simulink model "testFrame_PositionObserever"  (R2020b)
settings: Solver=FixedStepDiscrete  StartTime=0.0  StopTime=2  FixedStep=50e-6  RelTol=1e-3
undefined symbols (not defined in the file): BrkPoints, d_q_Voltage_Limiter_sat_neg, d_q_Voltage_Limiter_sat_pos, Ts
libraries: mcbcontrolslib x7, pid_lib x2, simulink x1
settings Model: DataDictionary=MotorControl.sldd  NumberOfSteps=10  Creator=unix  LastModifiedBy=unix
settings DebuggingCC: IntegerOverflowMsg=error  ParameterUnderflowMsg=error  IntegerSaturationMsg=error

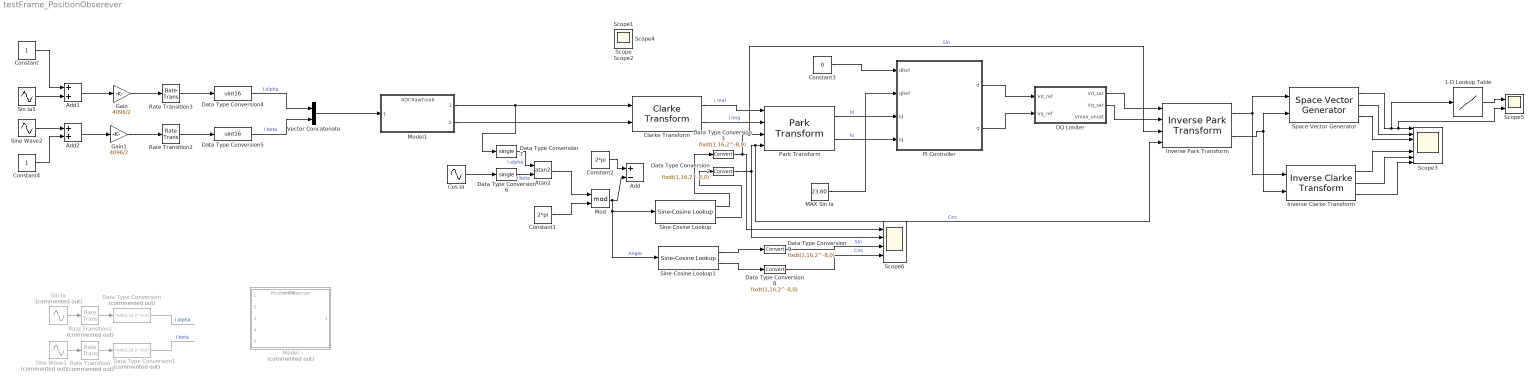
== system testFrame_PositionObserever ==
  1-D Lookup Table : Lookup_n-D  NumberOfTableDimensions=1  BreakpointsForDimension1=BrkPoints  Table=[0 250 500]  ExtrapMethod=Clip  InternalRulePriority=Speed  OutDataTypeStr=uint16  RndMeth=Simplest  SaturateOnIntegerOverflow=on  InputSameDT=on
  Add : Sum  Inputs=+-
  Add1 : Sum
  Add2 : Sum
  Atan2 : Trigonometry  Operator=atan2
  Clarke Transform : mcbcontrolslib/Clarke Transform  VariantControl=Variant2
  Constant : Constant
  Constant1 : Constant  Value=2*pi  OutDataTypeStr=Inherit: Inherit via back propagation
  Constant2 : Constant  Value=2*pi  OutDataTypeStr=Inherit: Inherit via back propagation
  Constant3 : Constant  Value=0  OutDataTypeStr=int8
  Constant4 : Constant
  Cos Ia : Sin  Amplitude=23.6  Frequency=100  Phase=pi/2  SampleTime=0
  DQ Limiter : Subsystem  AncestorBlock=mcbcontrolslib/DQ Limiter  mask(DQ Limiter){Vmax=5}
      mask prompts: Vmax "D-Q saturation limit:"
      mask help:
      | Implement saturation on reference dq voltages, with respect to phase voltage peak limit.
      |
      | The block accepts reference values of d and q axis voltages, and outputs corresponding saturated values along with unsaturated peak value to initiate field weakening control.
      |
      | Enter the phase voltage peak limit in the dialog box to initiate saturation.
      mask Help: eval('mcb.internal.helpview(''dqlimiter'')')
      mask Display: mcb.internal.drawIcons('DQ Limiter',1);
  Data Type Conversion : DataTypeConversion  Commented=on  OutDataTypeStr=fixdt(1,16,2^-8,0)
  Data Type Conversion1 : DataTypeConversion  Commented=on  OutDataTypeStr=fixdt(1,16,2^-8,0)
  Data Type Conversion{2..3,8..9} (4 alike) : DataTypeConversion  OutDataTypeStr=fixdt(1,16,2^-8,0)
  Data Type Conversion4 : DataTypeConversion  OutDataTypeStr=uint16
  Data Type Conversion5 : DataTypeConversion  OutDataTypeStr=uint16
  Data Type Conversion6 : DataTypeConversion  OutDataTypeStr=single
  Data Type Conversion7 : DataTypeConversion  OutDataTypeStr=single
  Gain : Gain  Gain=4096/2
  Gain1 : Gain  Gain=4096/2
  Inverse Clarke Transform : mcbcontrolslib/Inverse Clarke Transform
      settings: SourceProductBaseCode=MT
  Inverse Park Transform : mcbcontrolslib/Inverse Park Transform  AxisAlignment=D-axis
  MAX Sin Ia : Constant  Value=23.60  OutDataTypeStr=Inherit: Inherit via back propagation
  Mod : Math  Operator=mod  SaturateOnIntegerOverflow=on
  Model : ModelReference  Commented=on  ModelNameDialog=PositionObserver.slx  ModelReferenceVersion=3.3  EnablePortName=Enable  EnablePortStatesWhenEnabling=reset
  Model1 : ModelReference  ModelNameDialog=ADCRawToIab.slx  ModelReferenceVersion=3.3
  PI Controller : Subsystem
  Park Transform : mcbcontrolslib/Park Transform  AxisAlignment=D-axis
      settings: SourceProductBaseCode=MT
  Rate Transition : RateTransition  Commented=on  OutPortSampleTime=250e-6
  Rate Transition1 : RateTransition  Commented=on  OutPortSampleTime=250e-6
  Rate Transition2 : RateTransition  OutPortSampleTime=250e-6
  Rate Transition3 : RateTransition  OutPortSampleTime=250e-6
  Scope3 : Scope  NumInputPorts=7
  Scope5 : Scope  NumInputPorts=2
  Scope6 : Scope  NumInputPorts=4
  Sin Ia : Sin  Commented=on  Amplitude=25  Frequency=100  SampleTime=0
  Sin Ia1 : Sin  Frequency=100  SampleTime=0
  Sine Wave1 : Sin  Commented=on  Amplitude=25  Frequency=100  Phase=(2*pi)/3  SampleTime=0
  Sine Wave2 : Sin  Frequency=100  Phase=(2*pi)/3  SampleTime=0
  Sine-Cosine Lookup : mcbcontrolslib/Sine-Cosine Lookup  AngleInput=Radians  N_points=512
      settings: SourceProductBaseCode=MT
  Sine-Cosine Lookup1 : mcbcontrolslib/Sine-Cosine Lookup  AngleInput=Radians  N_points=512
      settings: SourceProductBaseCode=MT
  Space Vector Generator : mcbcontrolslib/Space Vector Generator
      settings: SourceProductBaseCode=MT
  Vector Concatenate : Concatenate
  Scope{,1..2,4} (4 alike) : Scope
  wires:
  Sine-Cosine Lookup/2 -> Data Type Conversion2/1
  Sine-Cosine Lookup/1 -> Data Type Conversion3/1
  Clarke Transform/1 -> Park Transform/1  "I real"
  Clarke Transform/2 -> Park Transform/2  "I img"
  Constant1/1 -> Mod/2
  Park Transform/1 -> PI Controller/3(Id)  "Id"
  Park Transform/2 -> PI Controller/4(Iq)  "Iq"
  Data Type Conversion2/1 -> Scope6/2, Inverse Park Transform/4, Park Transform/4  "Cos"
  Data Type Conversion3/1 -> Inverse Park Transform/3, Park Transform/3, Scope6/1  "Sin"
  Constant2/1 -> Add/1
  Constant3/1 -> PI Controller/1(dRef)
  MAX Sin Ia/1 -> PI Controller/2(qRef)
  PI Controller/1(d) -> DQ Limiter/1(Vd_ref)
  PI Controller/2(q) -> DQ Limiter/2(Vq_ref)
  Cos Ia/1 -> Data Type Conversion6/1
  Atan2/1 -> Mod/1
  Inverse Park Transform/1 -> Space Vector Generator/1, Inverse Clarke Transform/1
  Inverse Park Transform/2 -> Space Vector Generator/2, Inverse Clarke Transform/2
  Inverse Clarke Transform/1 -> Scope3/5
  Inverse Clarke Transform/2 -> Scope3/6
  Inverse Clarke Transform/3 -> Scope3/7
  Space Vector Generator/1 -> 1-D Lookup Table/1, Scope5/2, Scope3/1
  Space Vector Generator/2 -> Scope3/2
  Space Vector Generator/3 -> Scope3/3
  1-D Lookup Table/1 -> Scope5/1
  Rate Transition2/1 -> Data Type Conversion5/1
  Sine Wave2/1 -> Add2/1
  Rate Transition3/1 -> Data Type Conversion4/1
  Sin Ia1/1 -> Add1/2
  Gain/1 -> Rate Transition3/1
  Add1/1 -> Gain/1
  Constant/1 -> Add1/1
  Data Type Conversion4/1 -> Vector Concatenate/1  "I alpha"
  Data Type Conversion5/1 -> Vector Concatenate/2  "I beta"
  Vector Concatenate/1 -> Model1/1
  Model1/1 -> Data Type Conversion7/1, Clarke Transform/1
  Model1/2 -> Clarke Transform/2
  Constant4/1 -> Add2/2
  Add2/1 -> Gain1/1
  Gain1/1 -> Rate Transition2/1
  Data Type Conversion/1 -> ?  "I alpha"
  Sine Wave1/1 -> Rate Transition/1
  Data Type Conversion1/1 -> ?  "I beta"
  Rate Transition1/1 -> Data Type Conversion/1
  Rate Transition/1 -> Data Type Conversion1/1
  Sin Ia/1 -> Rate Transition1/1
  Data Type Conversion6/1 -> Atan2/2  "I beta"
  Data Type Conversion7/1 -> Atan2/1  "I alpha"
  DQ Limiter/1(Vd_sat) -> Inverse Park Transform/1
  DQ Limiter/2(Vq_sat) -> Inverse Park Transform/2
  Mod/1 -> Sine-Cosine Lookup1/1, Sine-Cosine Lookup/1, Add/2  "Angle"
  Sine-Cosine Lookup1/1 -> Data Type Conversion9/1
  Sine-Cosine Lookup1/2 -> Data Type Conversion8/1
  Data Type Conversion8/1 -> Scope6/4  "Cos"
  Data Type Conversion9/1 -> Scope6/3  "Sin"

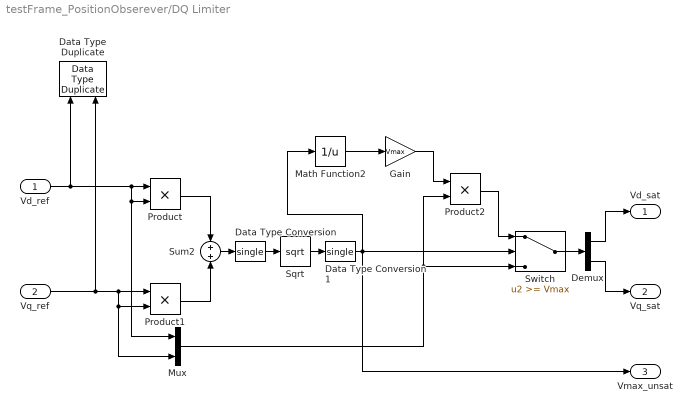
== system testFrame_PositionObserever/DQ Limiter ==
  Vd_ref : Inport
  Vq_ref : Inport  Port=2
  Data Type Duplicate : DataTypeDuplicate
  Data Type Conversion : DataTypeConversion  OutDataTypeStr=single
  Data Type Conversion1 : DataTypeConversion  OutDataTypeStr=single
  Demux : Demux  Outputs=2
  Gain : Gain  Gain=Vmax  OutDataTypeStr=Inherit: Same as input
  Math Function2 : Math  Operator=reciprocal  SignedPower=on  RndMeth=Simplest
  Mux : Mux  Inputs=2
  Product : Product  RndMeth=Simplest  OutDataTypeStr=Inherit: Same as first input
  Product1 : Product  RndMeth=Simplest  OutDataTypeStr=Inherit: Same as first input
  Product2 : Product  OutDataTypeStr=Inherit: Same as first input
  Sqrt : Sqrt  IntermediateResultsDataTypeStr=Inherit: Inherit from input  SaturateOnIntegerOverflow=on
  Sum2 : Sum  OutDataTypeStr=Inherit: Same as first input
  Switch : Switch  Threshold=Vmax  ZeroCross=off
  Vd_sat : Outport  VectorParamsAs1DForOutWhenUnconnected=off
  Vq_sat : Outport  Port=2  VectorParamsAs1DForOutWhenUnconnected=off
  Vmax_unsat : Outport  Port=3  VectorParamsAs1DForOutWhenUnconnected=off
  wires:
  Vd_ref/1 -> Data Type Duplicate/1, Product/1, Product/2, Mux/1
  Demux/1 -> Vd_sat/1
  Product1/1 -> Sum2/2
  Product/1 -> Sum2/1
  Sum2/1 -> Data Type Conversion/1
  Math Function2/1 -> Gain/1
  Mux/1 -> Product2/2, Switch/3
  Product2/1 -> Switch/1
  Switch/1 -> Demux/1
  Demux/2 -> Vq_sat/1
  Data Type Conversion1/1 -> Math Function2/1, Vmax_unsat/1, Switch/2
  Gain/1 -> Product2/1
  Vq_ref/1 -> Data Type Duplicate/2, Product1/1, Product1/2, Mux/2
  Data Type Conversion/1 -> Sqrt/1
  Sqrt/1 -> Data Type Conversion1/1

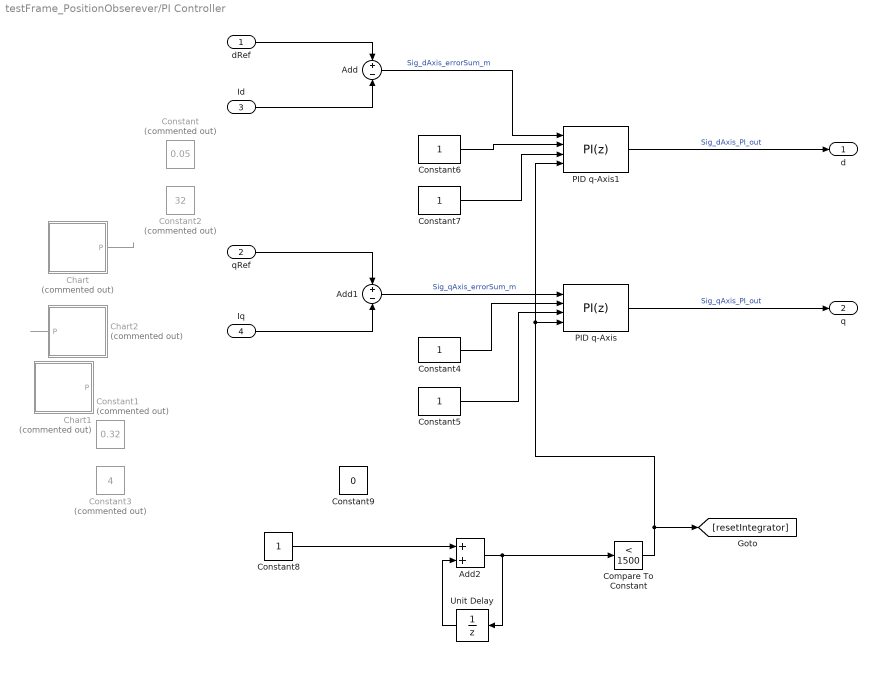
== system testFrame_PositionObserever/PI Controller ==
  dRef : Inport
  qRef : Inport  Port=2
  Id : Inport  Port=3
  Iq : Inport  Port=4
  Add : Sum  Inputs=+|-
  Add1 : Sum  Inputs=+|-
  Add2 : Sum
  Chart : Stateflow chart  Commented=on  TreatAsAtomicUnit=on  SystemSampleTime=1000*Ts
  Chart1 : Stateflow chart  Commented=on  TreatAsAtomicUnit=on  SystemSampleTime=2000*Ts
  Chart2 : Stateflow chart  Commented=on  TreatAsAtomicUnit=on  SystemSampleTime=100000*Ts
  Compare To Constant : simulink/Logic and Bit Operations/Compare To Constant  relop=<  const=1500  OutDataTypeStr=boolean
  Constant : Constant  Commented=on  Value=0.05  OutDataTypeStr=fixdt(1,16,2^-7,0)
  Constant1 : Constant  Commented=on  Value=0.32  OutDataTypeStr=fixdt(1,8,2^-7,0)
  Constant2 : Constant  Commented=on  Value=32  OutDataTypeStr=fixdt(1,8,2^-1,0)
  Constant3 : Constant  Commented=on  Value=4  OutDataTypeStr=fixdt(1,8,2^-1,0)
  Constant{4..7} (4 alike) : Constant  OutDataTypeStr=fixdt(1,16,2^-5,0)
  Constant8 : Constant
  Constant9 : Constant  Value=0  OutDataTypeStr=boolean
  PID q-Axis : pid_lib/PID Controller  Controller=PI  Form=Parallel  TimeDomain=Discrete-time  UseExternalTs=off  SampleTime=-1  IntegratorMethod=Forward Euler  FilterMethod=Forward Euler  ControllerParametersSource=external  P=0  I=0  D=0  UseFilter=on  N=100  TunerSelectOption=Transfer Function Based (PID Tuner App)  InitialConditionSource=internal  InitialConditionForIntegrator=0  InitialConditionForFilter=0  DifferentiatorICPrevScaledInput=0  ExternalReset=level  TrackingMode=off  Kt=1  LimitOutput=on  SatLimitsSource=internal  UpperSaturationLimit=d_q_Voltage_Limiter_sat_pos  LowerSaturationLimit=d_q_Voltage_Limiter_sat_neg  LinearizeAsGain=off  AntiWindupMode=clamping  Kb=10  PGainOutDataTypeStr=fixdt(1,16,2^-8,0)  PProdOutDataTypeStr=fixdt(1,16,2^-8,0)  POutMin=[]  POutMax=[]  IGainOutDataTypeStr=fixdt(1,16,2^-8,0)  IProdOutDataTypeStr=fixdt(1,16,2^-8,0)  IOutMin=[]  IOutMax=[]  DOutMin=[]  DOutMax=[]  NOutMin=[]  NOutMax=[]  SumOutDataTypeStr=fixdt(1,16,2^-8,0)  SumOutMin=[]  SumOutMax=[]  SaturationOutMin=[]  SaturationOutMax=[]  PParamMin=[]  PParamMax=[]  IParamMin=[]  IParamMax=[]  DParamMin=[]  DParamMax=[]  NParamMin=[]  NParamMax=[]  KbParamMin=[]  KbParamMax=[]  KtParamMin=[]  KtParamMax=[]  KbOutMin=[]  KbOutMax=[]  KtOutMin=[]  KtOutMax=[]  IntegratorOutDataTypeStr=fixdt(1,16,2^-8,0)  IntegratorOutMin=[]  IntegratorOutMax=[]  FilterOutMin=[]  FilterOutMax=[]  SumI1OutMin=[]  SumI1OutMax=[]  SumI2OutMin=[]  SumI2OutMax=[]  SumI3OutMin=[]  SumI3OutMax=[]  SumI4OutMin=[]  SumI4OutMax=[]  SumDOutMin=[]  SumDOutMax=[]  SumAccumDataTypeStr=fixdt(1,16,2^-8,0)  DifferentiatorOutMin=[]  DifferentiatorOutMax=[]  FilterDiffOutCoefMin=[]  FilterDiffOutCoefMax=[]  ReciprocalOutMin=[]  ReciprocalOutMax=[]  SumDenOutMin=[]  SumDenOutMax=[]  SumNumOutMin=[]  SumNumOutMax=[]  DivideOutMin=[]  DivideOutMax=[]  UdiffTsProdOutMin=[]  UdiffTsProdOutMax=[]  NTsProdOutMin=[]  NTsProdOutMax=[]  UintegralTsProdOutMin=[]  UintegralTsProdOutMax=[]  UngainTsProdOutMin=[]  UngainTsProdOutMax=[]  IntegratorContinuousStateAttributes=''  IntegratorStateMustResolveToSignalObject=off  IntegratorRTWStateStorageClass=Auto  FilterContinuousStateAttributes=''  FilterStateMustResolveToSignalObject=off  FilterRTWStateStorageClass=Auto  ParallelPVariant=ExternalParameters  IdealPVariant=Disabled  IVariant=ExternalParameters  DVariant=Disabled  IntegratorVariant=Discrete  SatVariant=Enabled  AWVariant=DiscClampingParallel  PCopyVariant=Disabled  TRVariant=Disabled  FdbkBlocksVariant=Forward  IdealPFdbkVariant=Disabled  SatFdbkVariant=Disabled  DerivativeFilterVariant=Disabled  NVariant=Disabled  NCopyVariant=Disabled_SignalSpec  FilterICVariant=Disabled  IntegratorICVariant=InternalICs  ExternalResetVariant=ExternalReset  TRSumVariant=Passthrough  SumFdbkVariant=Disabled  SumVariant=Sum_PI  TsampFilterVariant=InternalTs  TsampNgainVariant=Passthrough  TsampIntegralVariant=Passthrough  ExternalSaturationOutDataTypeStr=Inherit: Same as second input
  PID q-Axis1 : pid_lib/PID Controller  Controller=PI  Form=Parallel  TimeDomain=Discrete-time  UseExternalTs=off  SampleTime=-1  IntegratorMethod=Forward Euler  FilterMethod=Forward Euler  ControllerParametersSource=external  P=0  I=0  D=0  UseFilter=on  N=100  TunerSelectOption=Transfer Function Based (PID Tuner App)  ZeroCross=off  InitialConditionSource=internal  InitialConditionForIntegrator=0  InitialConditionForFilter=0  DifferentiatorICPrevScaledInput=0  ExternalReset=level  TrackingMode=off  Kt=1  LimitOutput=on  SatLimitsSource=internal  UpperSaturationLimit=d_q_Voltage_Limiter_sat_pos  LowerSaturationLimit=d_q_Voltage_Limiter_sat_neg  LinearizeAsGain=off  AntiWindupMode=clamping  Kb=10  PGainOutDataTypeStr=fixdt(1,16,2^-8,0)  PProdOutDataTypeStr=fixdt(1,16,2^-8,0)  POutMin=[]  POutMax=[]  IGainOutDataTypeStr=fixdt(1,16,2^-8,0)  IProdOutDataTypeStr=fixdt(1,16,2^-8,0)  IOutMin=[]  IOutMax=[]  DOutMin=[]  DOutMax=[]  NOutMin=[]  NOutMax=[]  SumOutDataTypeStr=fixdt(1,16,2^-8,0)  SumOutMin=[]  SumOutMax=[]  SaturationOutMin=[]  SaturationOutMax=[]  PParamMin=[]  PParamMax=[]  IParamMin=[]  IParamMax=[]  DParamMin=[]  DParamMax=[]  NParamMin=[]  NParamMax=[]  KbParamMin=[]  KbParamMax=[]  KtParamMin=[]  KtParamMax=[]  KbOutMin=[]  KbOutMax=[]  KtOutMin=[]  KtOutMax=[]  IntegratorOutDataTypeStr=fixdt(1,16,2^-8,0)  IntegratorOutMin=[]  IntegratorOutMax=[]  FilterOutMin=[]  FilterOutMax=[]  SumI1OutMin=[]  SumI1OutMax=[]  SumI2OutMin=[]  SumI2OutMax=[]  SumI3OutMin=[]  SumI3OutMax=[]  SumI4OutMin=[]  SumI4OutMax=[]  SumDOutMin=[]  SumDOutMax=[]  SumAccumDataTypeStr=fixdt(1,16,2^-8,0)  DifferentiatorOutMin=[]  DifferentiatorOutMax=[]  FilterDiffOutCoefMin=[]  FilterDiffOutCoefMax=[]  ReciprocalOutMin=[]  ReciprocalOutMax=[]  SumDenOutMin=[]  SumDenOutMax=[]  SumNumOutMin=[]  SumNumOutMax=[]  DivideOutMin=[]  DivideOutMax=[]  UdiffTsProdOutMin=[]  UdiffTsProdOutMax=[]  NTsProdOutMin=[]  NTsProdOutMax=[]  UintegralTsProdOutMin=[]  UintegralTsProdOutMax=[]  UngainTsProdOutMin=[]  UngainTsProdOutMax=[]  IntegratorContinuousStateAttributes=''  IntegratorStateMustResolveToSignalObject=off  IntegratorRTWStateStorageClass=Auto  FilterContinuousStateAttributes=''  FilterStateMustResolveToSignalObject=off  FilterRTWStateStorageClass=Auto  ParallelPVariant=ExternalParameters  IdealPVariant=Disabled  IVariant=ExternalParameters  DVariant=Disabled  IntegratorVariant=Discrete  SatVariant=Enabled  AWVariant=DiscClampingParallel  PCopyVariant=Disabled  TRVariant=Disabled  FdbkBlocksVariant=Forward  IdealPFdbkVariant=Disabled  SatFdbkVariant=Disabled  DerivativeFilterVariant=Disabled  NVariant=Disabled  NCopyVariant=Disabled_SignalSpec  FilterICVariant=Disabled  IntegratorICVariant=InternalICs  ExternalResetVariant=ExternalReset  TRSumVariant=Passthrough  SumFdbkVariant=Disabled  SumVariant=Sum_PI  TsampFilterVariant=InternalTs  TsampNgainVariant=Passthrough  TsampIntegralVariant=Passthrough  ExternalSaturationOutDataTypeStr=Inherit: Same as second input
  Unit Delay : UnitDelay  SampleTime=-1  HasFrameUpgradeWarning=on
  d : Outport
  q : Outport  Port=2
  wires:
  dRef/1 -> Add/1
  qRef/1 -> Add1/1
  Iq/1 -> Add1/2
  PID q-Axis/1 -> q/1  "Sig_qAxis_PI_out"
  PID q-Axis1/1 -> d/1  "Sig_dAxis_PI_out"
  Id/1 -> Add/2
  Add1/1 -> PID q-Axis/1  "Sig_qAxis_errorSum_m"
  Chart/1(P) -> ?
  Chart2/1(P) -> ?
  Constant5/1 -> PID q-Axis/3
  Constant4/1 -> PID q-Axis/2
  Add/1 -> PID q-Axis1/1  "Sig_dAxis_errorSum_m"
  Constant6/1 -> PID q-Axis1/2
  Constant7/1 -> PID q-Axis1/3
  Constant8/1 -> Add2/1
  Add2/1 -> Unit Delay/1, Compare To Constant/1
  Unit Delay/1 -> Add2/2
  Compare To Constant/1 -> [resetIntegrator], PID q-Axis1/4, PID q-Axis/4

== stateflow chart testFrame_PositionObserever/PI Controller/Chart1 ==
  (default) -> (junction 6) : /* P Value ++ */
  (junction 6) -> (junction 19) [order 1] : [P==0]{P=0.00;}
  (junction 6) -> (junction 17) [order 2]
  (junction 19) -> (junction 17)
  (junction 17) -> (junction 24) [order 2]
  (junction 17) -> (junction 8) [order 1] : {P+=0.1;}
  (junction 8) -> (junction 11) [order 2] : [P<=5]
  (junction 11) -> (junction 13)
  (junction 8) -> (junction 9) [order 1] : [P>5]{P=5;}
  (junction 9) -> (junction 13)
  data: P output double

== stateflow chart testFrame_PositionObserever/PI Controller/Chart ==
  (default) -> (junction 6) : /* P Value ++ */
  (junction 6) -> (junction 8) : {P+=0.001;}
  (junction 8) -> (junction 11) [order 2] : [P<=0]
  (junction 11) -> (junction 13)
  (junction 8) -> (junction 9) [order 1] : [P>0]{P=0.02;}
  (junction 9) -> (junction 13)
  data: P output double

== stateflow chart testFrame_PositionObserever/PI Controller/Chart2 ==
  (default) -> (junction 6) : /* P Value ++ */
  (junction 6) -> (junction 8) : {P+=1;}
  (junction 8) -> (junction 11) [order 2] : [P<=0]
  (junction 11) -> (junction 13)
  (junction 8) -> (junction 9) [order 1] : [P>0]{P=4;}
  (junction 9) -> (junction 13)
  data: P output double
